simulink model "MassaMollaLineare"  (R2022b)
settings: Solver=VariableStepAuto  StartTime=0.0  StopTime=20  RelTol=1e-3
values from neighbouring files (symbols this model uses):
  A = [0 1; -k/M -h/M]    [MassaMollaNonLineare.m]
  B = [0; 1/M]    [MassaMollaNonLineare.m]
  C = [1 0]    [MassaMollaNonLineare.m]
  D = 0    [MassaMollaNonLineare.m]
  x0 = [0; 0]    [MassaMollaNonLineare.m]
settings Model: Creator=TAWADROS  LastModifiedBy=TAWADROS

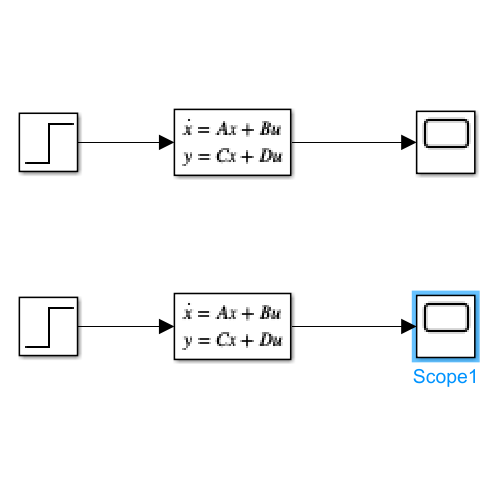
[thumbnail: Simulink's stored preview of the top-level diagram]
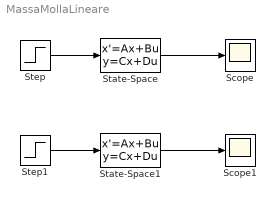
== system MassaMollaLineare ==
  Scope : Scope
  Scope1 : Scope
  State-Space : StateSpace  A=A  B=B  C=C  D=D  InitialCondition=x0
  State-Space1 : StateSpace  A=A  B=B  C=C  D=D  InitialCondition=x0
  Step : Step  SampleTime=0
  Step1 : Step  After=0.1  SampleTime=0  VectorParams1D=off  ZeroCross=off
  wires:
  Step/1 -> State-Space/1
  State-Space/1 -> Scope/1
  Step1/1 -> State-Space1/1
  State-Space1/1 -> Scope1/1
